simulink model "scheme1_sim"  (R2019b)
settings: Solver=ode4  StartTime=0.0  StopTime=Tsim  FixedStep=0.1  RelTol=1e-3
values from neighbouring files (symbols this model uses):
  Kd = 1.6797    [matlab_script.m]
  Ki = 0.5372    [matlab_script.m]
  Kp = 1.4968    [matlab_script.m]
  refmag = xxxx    [matlab_script.m]
settings Model: Creator=biannic  LastModifiedBy=biannic
settings DataIOCC: ReturnWorkspaceOutputs=off

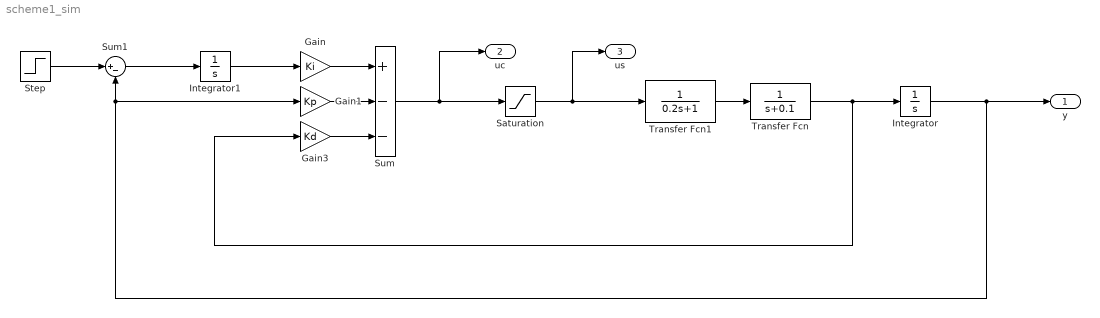
== system scheme1_sim ==
  Gain : Gain  Gain=Ki
  Gain1 : Gain  Gain=Kp
  Gain3 : Gain  Gain=Kd
  Integrator : Integrator
  Integrator1 : Integrator
  Saturation : Saturate  UpperLimit=0.1  LowerLimit=-0.1
  Step : Step  Time=0  After=refmag  SampleTime=0
  Sum : Sum  Inputs=+--
  Sum1 : Sum  Inputs=|+-
  Transfer Fcn : TransferFcn  Denominator=[1 0.1]
  Transfer Fcn1 : TransferFcn  Denominator=[0.2 1]
  y : Outport
  uc : Outport  Port=2
  us : Outport  Port=3
  wires:
  Step/1 -> Sum1/1
  Sum/1 -> Saturation/1, uc/1
  Transfer Fcn/1 -> Integrator/1, Gain3/1
  Integrator/1 -> y/1, Gain1/1, Sum1/2
  Sum1/1 -> Integrator1/1
  Saturation/1 -> Transfer Fcn1/1, us/1
  Transfer Fcn1/1 -> Transfer Fcn/1
  Gain/1 -> Sum/1
  Integrator1/1 -> Gain/1
  Gain1/1 -> Sum/2
  Gain3/1 -> Sum/3
